simulink model "StateFeedback2"  (R2018b)
settings: Solver=VariableStepAuto  StartTime=0.0  StopTime=12  RelTol=1e-3
settings Model: Creator=imi  LastModifiedBy=MJAHMADEE
settings SFSimCC: SimUseLocalCustomCode=off
settings RTWCC: RTWUseLocalCustomCode=off
settings CodeAppCC: StateflowObjectComments=on

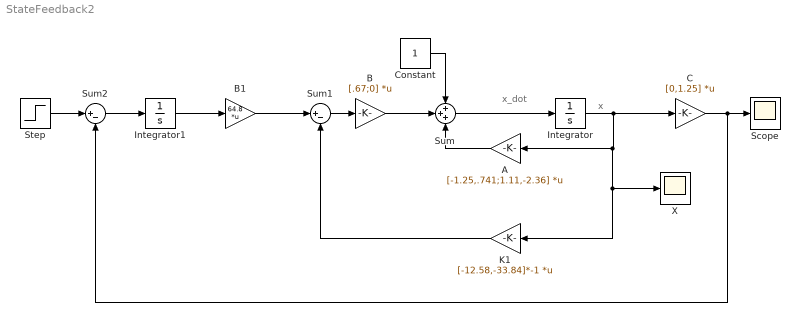
== system StateFeedback2 ==
  note: x
  note: x_dot
  A : Gain  Gain=[-1.25,.741;1.11,-2.36]  Multiplication=Matrix(K*u)
  B : Gain  Gain=[.67;0]  Multiplication=Matrix(K*u)
  B1 : Gain  Gain=64.8  Multiplication=Matrix(K*u)
  C : Gain  Gain=[0,1.25]  Multiplication=Matrix(K*u)
  Constant : Constant
  Integrator : Integrator  InitialCondition=[0;0]
  Integrator1 : Integrator
  K1 : Gain  Gain=[-12.58,-33.84]*-1  Multiplication=Matrix(K*u)
  Scope : Scope
  Step : Step  SampleTime=0
  Sum : Sum  Inputs=+++
  Sum1 : Sum  Inputs=|+-
  Sum2 : Sum  Inputs=|+-
  X : Scope
  wires:
  Sum/1 -> Integrator/1
  Integrator/1 -> C/1, X/1, K1/1, A/1
  Sum1/1 -> B/1
  K1/1 -> Sum1/2
  C/1 -> Sum2/2, Scope/1
  Step/1 -> Sum2/1
  Sum2/1 -> Integrator1/1
  B1/1 -> Sum1/1
  Integrator1/1 -> B1/1
  A/1 -> Sum/3
  B/1 -> Sum/2
  Constant/1 -> Sum/1
